simulink model "Three_Phase_Inverter_cricuit_plus_VFD"  (R2018b)
settings: Solver=VariableStepAuto  StartTime=0.0  StopTime=10.0  RelTol=1e-3
libraries: simulink x3, powerlib x2, powerlib_meascontrol x1
settings Model: Creator=pc  LastModifiedBy=pc

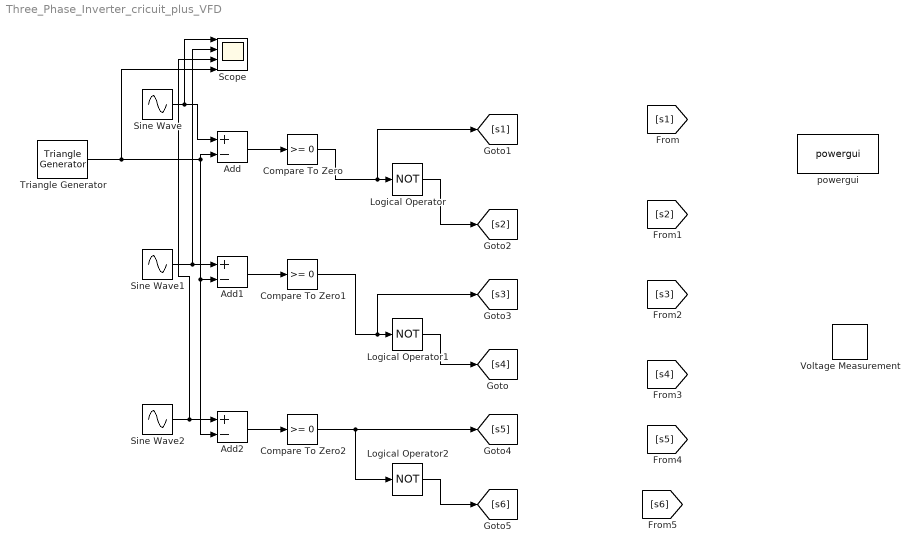
== system Three_Phase_Inverter_cricuit_plus_VFD ==
  Add : Sum  Inputs=+-
  Add1 : Sum  Inputs=+-
  Add2 : Sum  Inputs=+-
  Compare To Zero : simulink/Logic and Bit Operations/Compare To Zero  relop=>=  OutDataTypeStr=boolean
  Compare To Zero1 : simulink/Logic and Bit Operations/Compare To Zero  relop=>=  OutDataTypeStr=boolean
  Compare To Zero2 : simulink/Logic and Bit Operations/Compare To Zero  relop=>=  OutDataTypeStr=boolean
  Logical Operator : Logic  Operator=NOT  AllPortsSameDT=off  OutDataTypeStr=boolean
  Logical Operator1 : Logic  Operator=NOT  AllPortsSameDT=off  OutDataTypeStr=boolean
  Logical Operator2 : Logic  Operator=NOT  AllPortsSameDT=off  OutDataTypeStr=boolean
  Scope : Scope  NumInputPorts=4
  Sine Wave : Sin  Frequency=2*pi*50  SampleTime=0
  Sine Wave1 : Sin  Frequency=2*pi*50  Phase=2*pi/3  SampleTime=0
  Sine Wave2 : Sin  Frequency=2*pi*50  Phase=4*pi/3  SampleTime=0
  Triangle Generator : powerlib_meascontrol/Pulse & Signal Generators/Triangle Generator  Freq=1e3  Phase=180  Ts=0
  Voltage Measurement : powerlib/Measurements/Voltage Measurement  PhasorSimulation=off  OutputType=Complex  PSBequivalent=0
  powergui : powerlib/powergui  Priority=1  SimulationMode=Continuous  SampleTime=50e-6  frequency=60  Iterations=50  frequencyindice=60  Pbase=100e6  ErrMax=1e-4  UnitsV=kV  UnitsW=MW  buscounter=0  FunctionMessages=off  echomessages=off  EnableUseOfTLC=off  CurrentSourceSwitches=off  DisableSnubberDevices=off  DisableRonSwitches=off  DisableVfSwitches=off  DisplayEquations=off  SolverType=Tustin/Backward Euler (TBE)  Interpol=off  ExternalGateDelay=off  methode=off  Ts=100  x0status=blocks  SPID=on  SwTol=0  HookPort=off  RestoreLinks=warning  ResistiveCurrentMeasurement=off  Frange=[0:2:500]  Ylog=off  Xlog=on  ShowGrid=off  save=off  variable=ZData  structure=0  ZoomFFT=off  StartTime=0.0  cycles=1  DisplayStyle=1  fundamental=60  FreqAxis=off  MaxFrequency=1000  frequencyindicesteady=1  RmsSteady=1  display=off
  wires:
  Sine Wave/1 -> Scope/1, Add/1
  Triangle Generator/1 -> Scope/4, Add2/2, Add1/2, Add/2
  Sine Wave1/1 -> Scope/2, Add1/1
  Sine Wave2/1 -> Scope/3, Add2/1
  Add/1 -> Compare To Zero/1
  Add1/1 -> Compare To Zero1/1
  Add2/1 -> Compare To Zero2/1
  Compare To Zero/1 -> [s1], Logical Operator/1
  Compare To Zero1/1 -> [s3], Logical Operator1/1
  Compare To Zero2/1 -> [s5], Logical Operator2/1
  Logical Operator/1 -> [s2]
  Logical Operator1/1 -> [s4]
  Logical Operator2/1 -> [s6]
